simulink model "kontr_velocity"  (R2024a)
settings: Solver=VariableStepAuto  StartTime=0.0  StopTime=3  MaxStep=0.000001  RelTol=1e-3
settings Model: Creator=volko  LastModifiedBy=volko
settings RTWCC: GPUComputeCapability=3.5

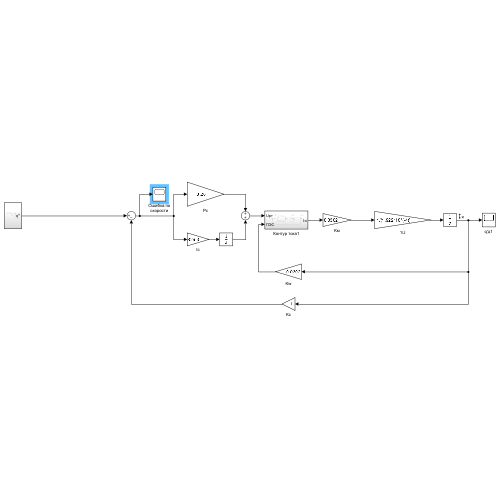
[thumbnail: Simulink's stored preview of the top-level diagram]
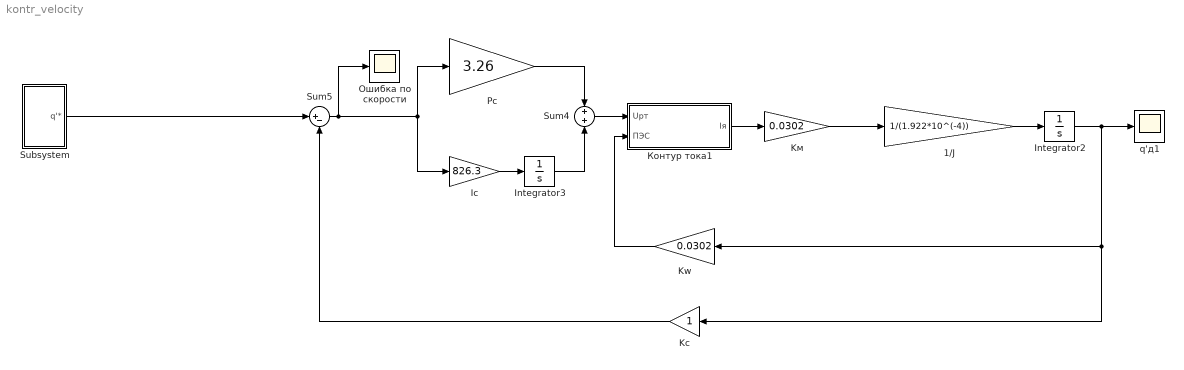
== system kontr_velocity ==
  1/J : Gain  Gain=1/(1.922*10^(-4))
  Integrator2 : Integrator
  Integrator3 : Integrator
  Iс : Gain  Gain=826.3
  Kw : Gain  Gain=0.0302
  Kм : Gain  Gain=0.0302
  Kс : Gain
  Pс : Gain  Gain=3.26
  Subsystem : Subsystem
  Sum4 : Sum
  Sum5 : Sum  Inputs=|+-
  q'д1 : Scope
  Контур тока1 : Subsystem
  Ошибка по скорости : Scope
  wires:
  Sum5/1 -> Ошибка по скорости/1, Pс/1, Iс/1
  Pс/1 -> Sum4/1
  Sum4/1 -> Контур тока1/1(Uрт)
  Kс/1 -> Sum5/2
  Iс/1 -> Integrator3/1
  Kw/1 -> Контур тока1/2(ПЭС)
  Integrator3/1 -> Sum4/2
  Integrator2/1 -> q'д1/1, Kс/1, Kw/1
  1/J/1 -> Integrator2/1
  Контур тока1/1(Iя) -> Kм/1
  Kм/1 -> 1/J/1
  Subsystem/1(q'*) -> Sum5/1

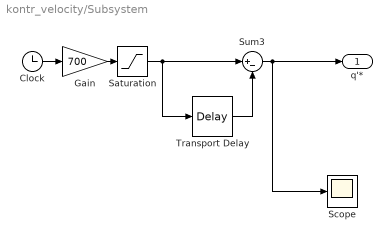
== system kontr_velocity/Subsystem ==
  Clock : Clock
  Gain : Gain  Gain=700
  Saturation : Saturate  UpperLimit=700  LowerLimit=0
  Scope : Scope
  Sum3 : Sum  Inputs=|+-
  Transport Delay : TransportDelay  DelayTime=1.5
  q'* : Outport
  wires:
  Clock/1 -> Gain/1
  Saturation/1 -> Sum3/1, Transport Delay/1
  Transport Delay/1 -> Sum3/2
  Gain/1 -> Saturation/1
  Sum3/1 -> q'*/1, Scope/1

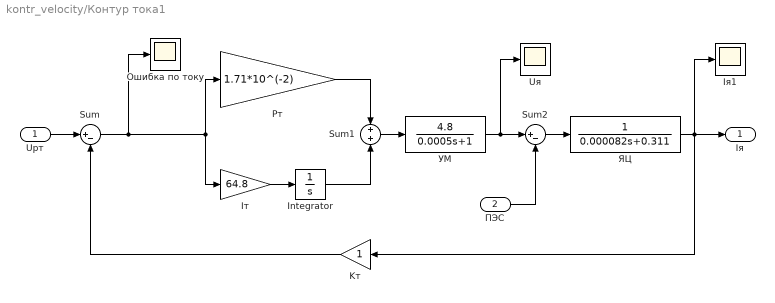
== system kontr_velocity/Контур тока1 ==
  Uрт : Inport
  ПЭС : Inport  Port=2
  Integrator : Integrator
  Iт : Gain  Gain=64.8
  Iя1 : Scope
  Kт : Gain
  Pт : Gain  Gain=1.71*10^(-2)
  Sum : Sum  Inputs=|+-
  Sum1 : Sum
  Sum2 : Sum  Inputs=|+-
  Uя : Scope
  Ошибка по току : Scope
  УМ : TransferFcn  Numerator=[4.8]  Denominator=[0.0005 1]
  ЯЦ : TransferFcn  Denominator=[0.000082 0.311]
  Iя : Outport
  wires:
  УМ/1 -> Sum2/1, Uя/1
  Integrator/1 -> Sum1/2
  Sum1/1 -> УМ/1
  Iт/1 -> Integrator/1
  Sum/1 -> Ошибка по току/1, Iт/1, Pт/1
  ЯЦ/1 -> Iя1/1, Iя/1, Kт/1
  Kт/1 -> Sum/2
  Pт/1 -> Sum1/1
  Uрт/1 -> Sum/1
  Sum2/1 -> ЯЦ/1
  ПЭС/1 -> Sum2/2
